simulink model "Model1"  (R2015a)
settings: Solver=ode45  StartTime=0.0  StopTime=10.0  RelTol=1e-3
settings Model: Creator=qiji  LastModifiedBy=qiji
settings DebuggingCC: UnderspecifiedInitializationDetection=Classic  MergeDetectMultiDrivingBlocksExec=none  SolverPrmCheckMsg=warning

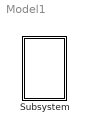
== system Model1 ==
  Subsystem : Subsystem

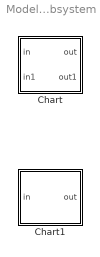
== system Model1/Subsystem ==
  Chart : Stateflow chart  TreatAsAtomicUnit=on
  Chart1 : Stateflow chart  TreatAsAtomicUnit=on

== stateflow chart Model1/Subsystem/Chart ==
  state A
    en:
    out = 0;
    out1 = 0;
  state B
    en:
    out = 1;
    out1 =1;
  A -> B : [in == 1]
  (default) -> A
  B -> A : [in==1]
  data: in input double; out output double; out1 output double; in1 input double

== stateflow chart Model1/Subsystem/Chart1 ==
  state A
    du:
    out = in
  (default) -> A
  data: in input double; out output double
